simulink model "gm_uz_JL_SigmaDelta_Interface"  (R2025a)
settings: Solver=FixedStepDiscrete  StartTime=0.0  StopTime=0.02  FixedStep=1e-08  RelTol=1e-3
undefined symbols (not defined in the file or in its folder): DiscIntNeverNeededParam
libraries: hdlstreaminglib x18, simulink x4, hdlsllib x2, simulink_extras x1
(part 2 of 2)

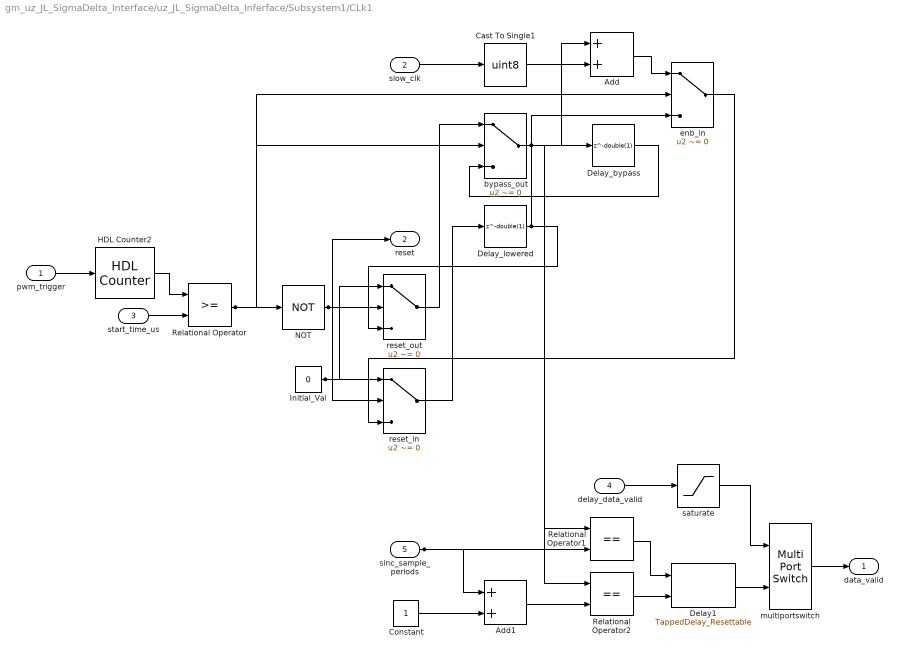
== system gm_uz_JL_SigmaDelta_Interface/uz_JL_SigmaDelta_Inferface/Subsystem1/CLk1 ==
  pwm_trigger : Inport  OutDataTypeStr=boolean  PortDimensions=1  SampleTime=1e-08
  slow_clk : Inport  Port=2  OutDataTypeStr=boolean  PortDimensions=1  SampleTime=1e-08
  start_time_us : Inport  Port=3  OutDataTypeStr=uint16  PortDimensions=1  SampleTime=1e-08
  delay_data_valid : Inport  Port=4  OutDataTypeStr=uint16  PortDimensions=1  SampleTime=1e-08
  sinc_sample_periods : Inport  Port=5  OutDataTypeStr=uint8  PortDimensions=1  SampleTime=1e-08
  Add : Sum  OutDataTypeStr=uint8  AccumDataTypeStr=uint8  SampleTime=1e-08
  Add1 : Sum  OutDataTypeStr=fixdt(0, 9, 0)  AccumDataTypeStr=fixdt(0, 9, 0)  SampleTime=1e-08
  Cast To Single1 : DataTypeConversion  OutDataTypeStr=uint8  SampleTime=1e-08  SaturateOnIntegerOverflow=off  RndMeth=Floor
  Constant : Constant  OutDataTypeStr=uint8  SampleTime=1e-08
  Delay1 : hdlstreaminglib/TappedDelay_Resettable  NumDelays=500  ResetTriggerType=level  DelayOrder=Newest  includeCurrent=on  samptime=-1  vinit=0
  Delay_bypass : Delay  DelayLength=double(1)  InitialCondition=0  SampleTime=1e-08
  Delay_lowered : Delay  DelayLength=double(1)  InitialCondition=0  SampleTime=1e-08
  HDL Counter2 : hdlsllib/Sources/HDL Counter  CountType=Free running  CountInit=1  CountStep=1  CountMax=25  CountFromType=Initial value  CountFrom=1  CountResetPort=on  CountLoadPort=off  CountEnbPort=off  CountDirPort=off  CountHitOutputPort=off  CountDataType=Unsigned  CountWordLen=16  CountFracLen=0  CountSampTime=1
  Initial_Val : Constant  Value=0  OutDataTypeStr=uint8  SampleTime=1e-08
  NOT : Logic  Operator=NOT  Inputs=1  AllPortsSameDT=off  OutDataTypeStr=boolean  SampleTime=1e-08
  Relational Operator : RelationalOperator  OutDataTypeStr=boolean  SampleTime=1e-08  InputSameDT=off
  Relational Operator1 : RelationalOperator  Operator===  OutDataTypeStr=boolean  SampleTime=1e-08  InputSameDT=off
  Relational Operator2 : RelationalOperator  Operator===  OutDataTypeStr=boolean  SampleTime=1e-08  InputSameDT=off
  bypass_out : Switch  Criteria=u2 ~= 0  Threshold=double(0)  OutDataTypeStr=uint8  SampleTime=1e-08  SaturateOnIntegerOverflow=off  InputSameDT=off
  enb_in : Switch  Criteria=u2 ~= 0  Threshold=double(0)  OutDataTypeStr=uint8  SampleTime=1e-08  SaturateOnIntegerOverflow=off  InputSameDT=off
  multiportswitch : MultiPortSwitch  DataPortOrder=Zero-based contiguous  Inputs=1  DiagnosticForDefault=None  zeroidx=on  SampleTime=1e-08  SaturateOnIntegerOverflow=off  InputSameDT=off
  reset_in : Switch  Criteria=u2 ~= 0  Threshold=double(0)  OutDataTypeStr=uint8  SampleTime=1e-08  SaturateOnIntegerOverflow=off  InputSameDT=off
  reset_out : Switch  Criteria=u2 ~= 0  Threshold=double(0)  OutDataTypeStr=uint8  SampleTime=1e-08  SaturateOnIntegerOverflow=off  InputSameDT=off
  saturate : Saturate  UpperLimit=double(500)  LowerLimit=double(0)  SampleTime=1e-08  OutDataTypeStr=uint16
  data_valid : Outport  SampleTime=1e-08
  reset : Outport  Port=2  SampleTime=1e-08
  wires:
  HDL Counter2/1 -> Relational Operator/1
  Add/1 -> enb_in/1
  pwm_trigger/1 -> HDL Counter2/1
  reset_out/1 -> bypass_out/1
  start_time_us/1 -> Relational Operator/2
  slow_clk/1 -> Cast To Single1/1
  Relational Operator/1 -> bypass_out/2, enb_in/2, NOT/1
  NOT/1 -> reset_out/2, reset_in/2, reset/1
  Initial_Val/1 -> reset_out/1, reset_in/1
  reset_in/1 -> Delay_lowered/1
  sinc_sample_periods/1 -> Relational Operator1/2, Add1/1
  enb_in/1 -> reset_in/3
  Constant/1 -> Add1/2
  Cast To Single1/1 -> Add/2
  bypass_out/1 -> Relational Operator2/1, Relational Operator1/1, Delay_bypass/1, Add/1
  Delay_lowered/1 -> reset_out/3, enb_in/3
  Add1/1 -> Relational Operator2/2
  Delay_bypass/1 -> bypass_out/3
  delay_data_valid/1 -> saturate/1
  Relational Operator1/1 -> Delay1/1
  Relational Operator2/1 -> Delay1/2
  saturate/1 -> multiportswitch/1
  Delay1/1 -> multiportswitch/2
  multiportswitch/1 -> data_valid/1
